simulink model "rDischargeDerate"  (R2024b)
settings: configuration reference "STM32H7_Config" (kept outside this file)
settings Model: DataDictionary=Master_Dictionary.sldd  EnableAccessToBaseWorkspace=off  Creator=torni  LastModifiedBy=William
settings ConfigSetRef: SourceName=STM32H7_Config

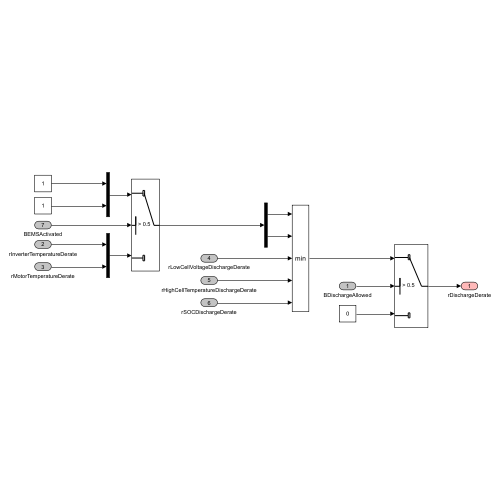
[thumbnail: Simulink's stored preview of the top-level diagram]
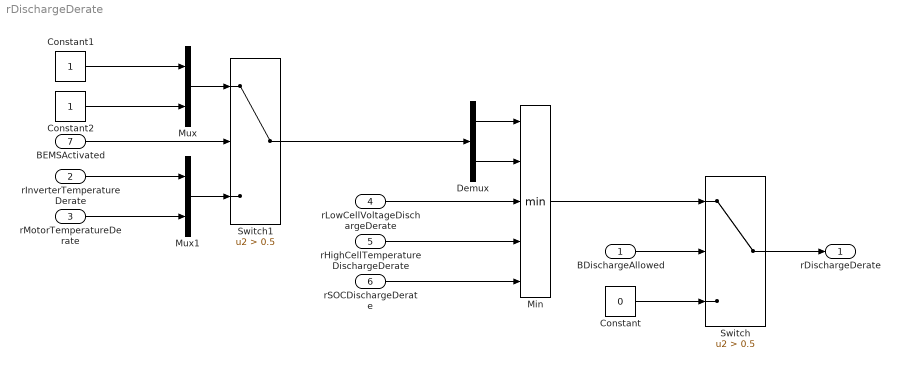
== system rDischargeDerate ==
  "BDischargeAllowed " : Inport  OutDataTypeStr=boolean
  rInverterTemperatureDerate : Inport  Port=2  OutDataTypeStr=double
  rMotorTemperatureDerate : Inport  Port=3  OutDataTypeStr=double
  rLowCellVoltageDischargeDerate : Inport  Port=4  OutDataTypeStr=double
  rHighCellTemperatureDischargeDerate : Inport  Port=5  OutDataTypeStr=double
  rSOCDischargeDerate : Inport  Port=6  OutDataTypeStr=double
  BEMSActivated : Inport  Port=7  OutDataTypeStr=boolean
  Constant : Constant  Value=0
  Constant1 : Constant
  Constant2 : Constant
  Demux : Demux  Outputs=2
  Min : MinMax  Inputs=5
  Mux : Mux  Inputs=2
  Mux1 : Mux  Inputs=2
  Switch : Switch  Criteria=u2 > Threshold  Threshold=0.5  SaturateOnIntegerOverflow=off  InputSameDT=off
  Switch1 : Switch  Criteria=u2 > Threshold  Threshold=0.5  SaturateOnIntegerOverflow=off  InputSameDT=off
  rDischargeDerate : Outport  OutDataTypeStr=double  VectorParamsAs1DForOutWhenUnconnected=off
  wires:
  Constant/1 -> Switch/3
  Min/1 -> Switch/1
  rInverterTemperatureDerate/1 -> Mux1/1
  rMotorTemperatureDerate/1 -> Mux1/2
  Switch/1 -> rDischargeDerate/1
  "BDischargeAllowed "/1 -> Switch/2
  rLowCellVoltageDischargeDerate/1 -> Min/3
  rSOCDischargeDerate/1 -> Min/5
  rHighCellTemperatureDischargeDerate/1 -> Min/4
  Constant1/1 -> Mux/1
  Constant2/1 -> Mux/2
  Demux/1 -> Min/1
  Demux/2 -> Min/2
  BEMSActivated/1 -> Switch1/2
  Mux/1 -> Switch1/1
  Mux1/1 -> Switch1/3
  Switch1/1 -> Demux/1
